simulink model "model_for_screen"  (R2024a)
settings: Solver=ode15s  StartTime=0.0  StopTime=0.25  FixedStep=1e-4  RelTol=1e-3
undefined symbols (not defined in the file): data, data_SL_Info, effort, effort_SL_Info, name, name_SL_Info, position, position_SL_Info, velocity, velocity_SL_Info, X, Y, Z
libraries: sm_lib x42, nesl_utility x14, ros2lib x6
(part 2 of 2)

== system model_for_screen/ROS Send message/Naming/Subsystem ==
  In1 : Inport
  Bus Assignment1 : BusAssignment  AssignedSignals=data,data_SL_Info.CurrentLength
  Constant3 : Constant  Value=0  OutDataTypeStr=Bus: SL_Bus_std_msgs_String
  Constant4 : Constant  Value=128  OutDataTypeStr=uint32
  String to ASCII : StringToASCII  OutputVectorSize=128
  Out1 : Outport
  wires:
  String to ASCII/1 -> Bus Assignment1/2
  Constant4/1 -> Bus Assignment1/3
  Constant3/1 -> Bus Assignment1/1
  Bus Assignment1/1 -> Out1/1
  In1/1 -> String to ASCII/1

== system model_for_screen/ROS Send message/Naming/Subsystem1 ==
  In1 : Inport
  Bus Assignment1 : BusAssignment  AssignedSignals=data,data_SL_Info.CurrentLength
  Constant3 : Constant  Value=0  OutDataTypeStr=Bus: SL_Bus_std_msgs_String
  Constant4 : Constant  Value=128  OutDataTypeStr=uint32
  String to ASCII : StringToASCII  OutputVectorSize=128
  Out1 : Outport
  wires:
  String to ASCII/1 -> Bus Assignment1/2
  Constant4/1 -> Bus Assignment1/3
  Constant3/1 -> Bus Assignment1/1
  Bus Assignment1/1 -> Out1/1
  In1/1 -> String to ASCII/1

== system model_for_screen/ROS Send message/Naming/Subsystem2 ==
  In1 : Inport
  Bus Assignment1 : BusAssignment  AssignedSignals=data,data_SL_Info.CurrentLength
  Constant3 : Constant  Value=0  OutDataTypeStr=Bus: SL_Bus_std_msgs_String
  Constant4 : Constant  Value=128  OutDataTypeStr=uint32
  String to ASCII : StringToASCII  OutputVectorSize=128
  Out1 : Outport
  wires:
  String to ASCII/1 -> Bus Assignment1/2
  Constant4/1 -> Bus Assignment1/3
  Constant3/1 -> Bus Assignment1/1
  Bus Assignment1/1 -> Out1/1
  In1/1 -> String to ASCII/1

== system model_for_screen/ROS Send message/Naming/Subsystem3 ==
  In1 : Inport
  Bus Assignment1 : BusAssignment  AssignedSignals=data,data_SL_Info.CurrentLength
  Constant3 : Constant  Value=0  OutDataTypeStr=Bus: SL_Bus_std_msgs_String
  Constant4 : Constant  Value=128  OutDataTypeStr=uint32
  String to ASCII : StringToASCII  OutputVectorSize=128
  Out1 : Outport
  wires:
  String to ASCII/1 -> Bus Assignment1/2
  Constant4/1 -> Bus Assignment1/3
  Constant3/1 -> Bus Assignment1/1
  Bus Assignment1/1 -> Out1/1
  In1/1 -> String to ASCII/1
